simulink model "LEDs"  (R2023b)
settings: Solver=FixedStepAuto  StartTime=0.0  StopTime=inf  RelTol=1e-3  EnableMultiTasking=on
libraries: arduinolib x6
settings Model: ExtModeTrigDuration=2  Creator=chaya  LastModifiedBy=chaya
settings OptimizationCC: EnhancedBackFolding=on  PassReuseOutputArgsAs=Individual arguments  ZeroExternalMemoryAtStartup=off  ZeroInternalMemoryAtStartup=off  MaxStackSize=64  OptimizeBlockOrder=speed  DifferentSizesBufferReuse=on  OptimizationCustomize=off  EfficientTunableParamExpr=on
settings DebuggingCC: ParameterTunabilityLossMsg=error
settings HardwareCC: ProdBitPerInt=16  ProdBitPerPointer=16  ProdBitPerSizeT=16  ProdBitPerPtrDiffT=16  ProdLargestAtomicFloat=None  ProdWordSize=8  ProdHWDeviceType=Atmel->AVR  UseEmbeddedCoderFeatures=off  UseSimulinkCoderFeatures=off
settings SFSimCC: MATLABDynamicMemAlloc=off
settings RTWCC: Description=Embedded Coder  SystemTargetFile=ert.tlc  HardwareBoard=Arduino Mega 2560  TemplateMakefile=ert_default_tmf  Toolchain=Arduino AVR  BuildConfiguration=Faster Runs
settings CodeAppCC: ForceParamTrailComments=on  IgnoreCustomStorageClasses=off  OperatorAnnotations=on  SimulinkDataObjDesc=on  SFDataObjDesc=on  InsertBlockDesc=on
settings ERTTargetCC: SupportContinuousTime=on  SupportNonInlinedSFcns=on  SupportVariableSizeSignals=on  ExtModeTransport=3  ExtModeStaticAlloc=on  ExtModeAutomaticAllocSize=off  ExtModeStaticAllocSize=2048  ExtModeMexFile=ext_xcp  ExtModeIntrfLevel=Level2 - Open

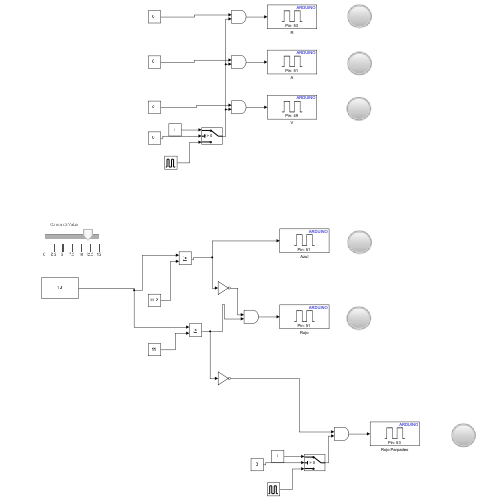
[thumbnail: Simulink's stored preview of the top-level diagram]
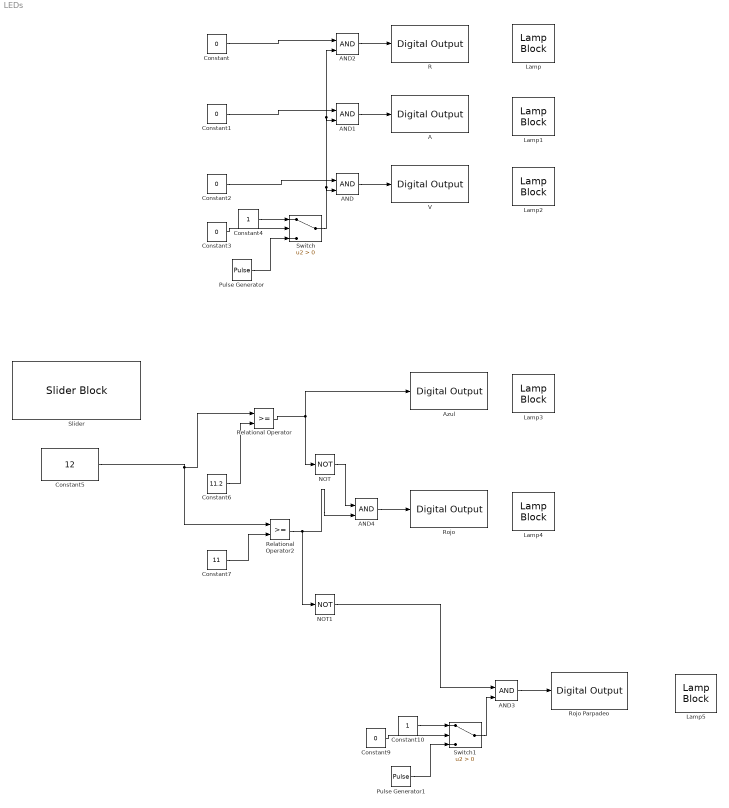
== system LEDs ==
  A : arduinolib/Digital Output  pinNumber=51  Direction=output  blockPlatform=arduino
  AND{,1..4} (5 alike) : Logic  IconShape=distinctive  AllPortsSameDT=off  OutDataTypeStr=boolean
  Azul : arduinolib/Digital Output  pinNumber=51  Direction=output  blockPlatform=arduino
  Constant{,1..3,9} (5 alike) : Constant  Value=0
  Constant10 : Constant
  Constant4 : Constant
  Constant5 : Constant  Value=12
  Constant6 : Constant  Value=11.2
  Constant7 : Constant  Value=11
  Lamp{,1..5} (6 alike) : LampBlock  LabelPosition=Hide
  NOT : Logic  Operator=NOT  IconShape=distinctive  AllPortsSameDT=off  OutDataTypeStr=boolean
  NOT1 : Logic  Operator=NOT  IconShape=distinctive  AllPortsSameDT=off  OutDataTypeStr=boolean
  Pulse Generator : DiscretePulseGenerator  PulseType=Time based  Period=1  PulseWidth=50
  Pulse Generator1 : DiscretePulseGenerator  PulseType=Time based  Period=1  PulseWidth=50
  R : arduinolib/Digital Output  pinNumber=53  Direction=output  blockPlatform=arduino
  Relational Operator : RelationalOperator  OutDataTypeStr=boolean  RndMeth=Simplest  InputSameDT=off
  Relational Operator2 : RelationalOperator  OutDataTypeStr=boolean  RndMeth=Simplest  InputSameDT=off
  Rojo : arduinolib/Digital Output  pinNumber=51  Direction=output  blockPlatform=arduino
  Rojo Parpadeo : arduinolib/Digital Output  pinNumber=53  Direction=output  blockPlatform=arduino
  Slider : SliderBlock  ScaleMax=15
  Switch : Switch  Criteria=u2 > Threshold  SaturateOnIntegerOverflow=off  InputSameDT=off
  Switch1 : Switch  Criteria=u2 > Threshold  SaturateOnIntegerOverflow=off  InputSameDT=off
  V : arduinolib/Digital Output  pinNumber=49  Direction=output  blockPlatform=arduino
  wires:
  AND1/1 -> A/1
  Constant/1 -> AND2/1
  AND2/1 -> R/1
  Constant1/1 -> AND1/1
  Constant4/1 -> Switch/1
  Constant2/1 -> AND/1
  Constant3/1 -> Switch/2
  Switch/1 -> AND2/2, AND1/2, AND/2
  Pulse Generator/1 -> Switch/3
  AND/1 -> V/1
  Constant5/1 -> Relational Operator2/1, Relational Operator/1
  Constant6/1 -> Relational Operator/2
  Relational Operator/1 -> NOT/1, Azul/1
  Constant7/1 -> Relational Operator2/2
  Relational Operator2/1 -> AND4/2, NOT1/1
  Pulse Generator1/1 -> Switch1/3
  NOT1/1 -> AND3/1
  Constant9/1 -> Switch1/2
  Constant10/1 -> Switch1/1
  Switch1/1 -> AND3/2
  AND3/1 -> Rojo Parpadeo/1
  AND4/1 -> Rojo/1
  NOT/1 -> AND4/1
